simulink library "aac"  (Simulink 8.1)
settings: Solver=ode45  StartTime=0.0  StopTime=10.0  RelTol=1e-3
undefined symbols (not defined in the file or in its folder): KJUD_BrakePreFillDelay_ms
libraries: hcu_lib x1
settings Model: Creator=xsellart  LastModifiedBy=tescamilla

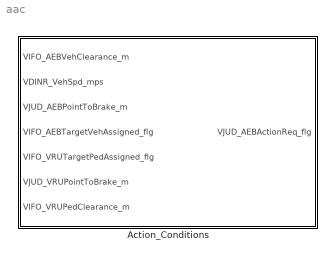
== system aac ==
  Action_Conditions : Subsystem

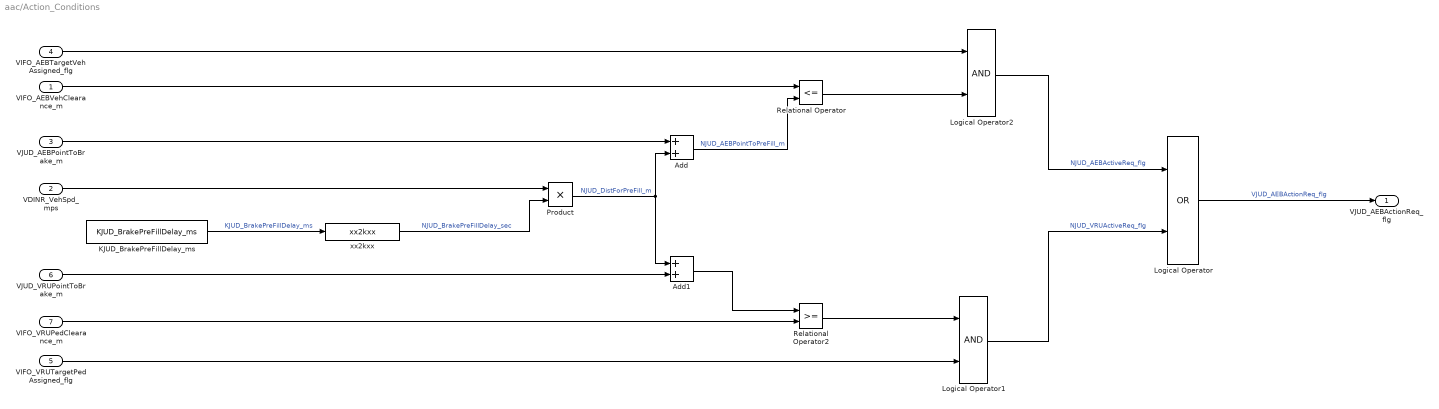
== system aac/Action_Conditions ==
  VIFO_AEBVehClearance_m : Inport
  VDINR_VehSpd_mps : Inport  Port=2
  VJUD_AEBPointToBrake_m : Inport  Port=3
  VIFO_AEBTargetVehAssigned_flg : Inport  Port=4
  VIFO_VRUTargetPedAssigned_flg : Inport  Port=5
  VJUD_VRUPointToBrake_m : Inport  Port=6
  VIFO_VRUPedClearance_m : Inport  Port=7
  Add : Sum
  Add1 : Sum
  KJUD_BrakePreFillDelay_ms : Constant  Value=KJUD_BrakePreFillDelay_ms
  Logical Operator : Logic  Operator=OR  AllPortsSameDT=off  OutDataTypeStr=boolean
  Logical Operator1 : Logic  AllPortsSameDT=off  OutDataTypeStr=boolean
  Logical Operator2 : Logic  AllPortsSameDT=off  OutDataTypeStr=boolean
  Product : Product
  Relational Operator : RelationalOperator  Operator=<=  OutDataTypeStr=boolean
  Relational Operator2 : RelationalOperator  OutDataTypeStr=boolean
  xx2kxx : hcu_lib/xx2kxx
  VJUD_AEBActionReq_flg : Outport
  wires:
  VJUD_AEBPointToBrake_m/1 -> Add/1
  Relational Operator/1 -> Logical Operator2/2
  VIFO_AEBVehClearance_m/1 -> Relational Operator/1
  Logical Operator/1 -> VJUD_AEBActionReq_flg/1  "VJUD_AEBActionReq_flg"
  VDINR_VehSpd_mps/1 -> Product/1
  KJUD_BrakePreFillDelay_ms/1 -> xx2kxx/1  "KJUD_BrakePreFillDelay_ms"
  Product/1 -> Add1/1, Add/2  "NJUD_DistForPreFill_m"
  Add/1 -> Relational Operator/2  "NJUD_AEBPointToPreFill_m"
  xx2kxx/1 -> Product/2  "NJUD_BrakePreFillDelay_sec"
  VIFO_AEBTargetVehAssigned_flg/1 -> Logical Operator2/1
  VJUD_VRUPointToBrake_m/1 -> Add1/2
  VIFO_VRUPedClearance_m/1 -> Relational Operator2/2
  Add1/1 -> Relational Operator2/1
  Relational Operator2/1 -> Logical Operator1/1
  Logical Operator2/1 -> Logical Operator/1  "NJUD_AEBActiveReq_flg"
  VIFO_VRUTargetPedAssigned_flg/1 -> Logical Operator1/2
  Logical Operator1/1 -> Logical Operator/2  "NJUD_VRUActiveReq_flg"
